simulink model "problem1"  (R2020b)
settings: Solver=VariableStepAuto  StartTime=0.0  StopTime=10.0  RelTol=1e-3
PreLoadFcn:
  | t=1:100;
  | F=2*sin(10*t);
  | K1=50;
  | b=50;
  | M1=100;
  | k12=1000;
  | M2=0.25;
settings Model: Creator=Sayan  LastModifiedBy=Sayan

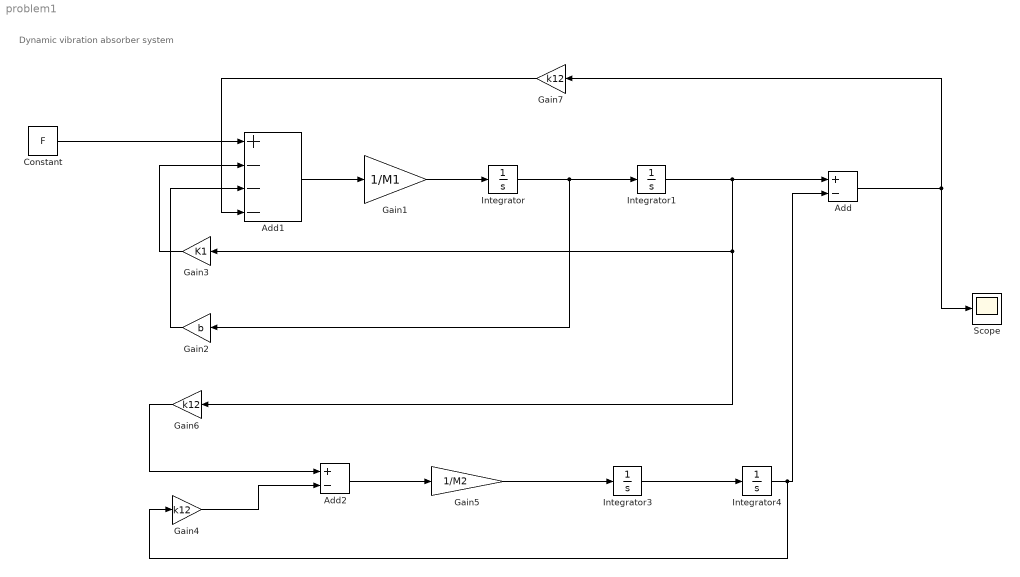
== system problem1 ==
  note: Dynamic vibration absorber system
  Add : Sum  Inputs=+-
  Add1 : Sum  Inputs=+---
  Add2 : Sum  Inputs=+-
  Constant : Constant  Value=F
  Gain1 : Gain  Gain=1/M1
  Gain2 : Gain  Gain=b
  Gain3 : Gain  Gain=K1
  Gain4 : Gain  Gain=k12
  Gain5 : Gain  Gain=1/M2
  Gain6 : Gain  Gain=k12
  Gain7 : Gain  Gain=k12
  Integrator{,1,3..4} (4 alike) : Integrator
  Scope : Scope
  wires:
  Gain2/1 -> Add1/3
  Gain5/1 -> Integrator3/1
  Integrator1/1 -> Add/1, Gain3/1, Gain6/1
  Add2/1 -> Gain5/1
  Integrator/1 -> Integrator1/1, Gain2/1
  Gain4/1 -> Add2/2
  Gain6/1 -> Add2/1
  Integrator3/1 -> Integrator4/1
  Integrator4/1 -> Add/2, Gain4/1
  Gain1/1 -> Integrator/1
  Gain7/1 -> Add1/4
  Add1/1 -> Gain1/1
  Add/1 -> Gain7/1, Scope/1
  Constant/1 -> Add1/1
  Gain3/1 -> Add1/2
